simulink model "Filtro_teste_potencia_constante_burrice"  (R2014b)
settings: Solver=ode45  StartTime=0.0  StopTime=0.015  MaxStep=1e-6  RelTol=1e-5
libraries: powerlib x15, powerlib_meascontrol x2, powerlib_extras x1, dsparch4 x1
settings Model: Creator=JPSOLIV  LastModifiedBy=JPSOLIV

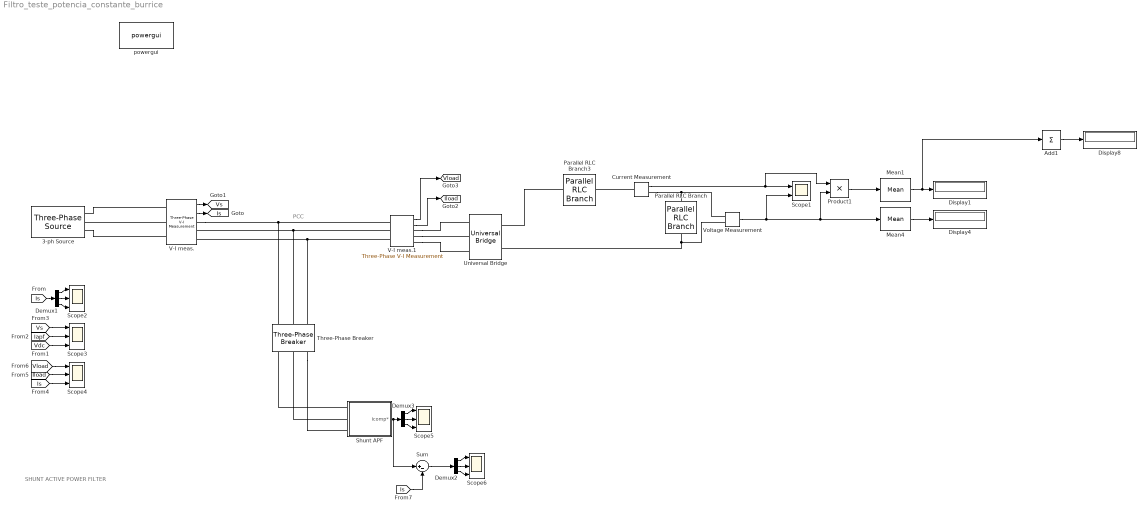
== system Filtro_teste_potencia_constante_burrice ==
  note: SHUNT ACTIVE POWER FILTER
  note: PCC
  3-ph Source : powerlib/Electrical Sources/Three-Phase Source  Voltage=115*sqrt(3)  PhaseAngle=0  Frequency=400  InternalConnection=Yg  SpecifyImpedance=off  Resistance=0.001  Inductance=1e-8  ShortCircuitLevel=100e6  BaseVoltage=25e3  XRratio=7  BusType=swing  Pref=0  Qref=0  Qmin=-inf  Qmax=inf
  Add1 : Sum  Inputs=+
  Current Measurement : powerlib/Measurements/Current Measurement  PhasorSimulation=off  OutputType=Complex  PSBequivalent=0
  Demux1 : Demux  Outputs=3
  Demux2 : Demux  Outputs=3
  Demux3 : Demux  Outputs=3
  Display1 : Display
  Display4 : Display
  Display8 : Display
  Mean1 : powerlib_meascontrol/Measurements/Mean  Freq=400  Vinit=0  Ts=0
  Mean4 : powerlib_meascontrol/Measurements/Mean  Freq=400  Vinit=0  Ts=0
  Parallel RLC Branch : powerlib/Elements/Parallel RLC Branch  LConnTagsString=a  RConnTagsString=__new0  BranchType=RC  Resistance=100  Inductance=1e-3  SetiL0=off  InitialCurrent=0  Capacitance=30e-6  Setx0=off  InitialVoltage=0  Measurements=None
  Parallel RLC Branch3 : powerlib/Elements/Parallel RLC Branch  LConnTagsString=a  RConnTagsString=__new0  BranchType=L  Resistance=1  Inductance=0.1e-3  SetiL0=off  InitialCurrent=0  Capacitance=30e-6  Setx0=off  InitialVoltage=0  Measurements=None
  Product1 : Product
  Scope1 : Scope  NumInputPorts=2
      settings: YMin=-20~0  YMax=160~600
  Scope{2..6} (5 alike) : Scope  NumInputPorts=3
      Scope2 settings: TimeRange=0.015  YMin=-2~-200~-50  YMax=12~50~200  SaveName=Isource  MaxDataPoints=500000
      Scope3 settings: TimeRange=0.015  YMin=-200~-10~-500  YMax=200~20~1500  SaveName=Vs_Iapf_Vdc  MaxDataPoints=500000
      Scope4 settings: TimeRange=0.015  YMin=-200~-200~-200  YMax=200~200~200  SaveName=Vs_Iapf_Vdc1  MaxDataPoints=500000
      Scope5 settings: TimeRange=0.015  YMin=-15~-50~-200  YMax=10~200~50  SaveName=Icomp  MaxDataPoints=500000
      Scope6 settings: TimeRange=0.015  YMin=-30~-30~-30  YMax=30~20~30  SaveName=Icomp1  MaxDataPoints=500000
  Shunt APF : Subsystem
  Sum : Sum  Inputs=|+-
  Three-Phase Breaker : powerlib/Elements/Three-Phase Breaker  InitialState=open  SwitchA=on  SwitchB=on  SwitchC=on  SwitchTimes=0.001  External=off  BreakerResistance=1e-6  SnubberResistance=1e6  SnubberCapacitance=inf  Measurements=None
  Universal Bridge : powerlib/Power Electronics/Universal Bridge  Arms=3  SnubberResistance=1e5  SnubberCapacitance=inf  Device=Diodes  Ron=1e-3  Lon=0  ForwardVoltages="[  0  0  ]"  ForwardVoltage=0  GTOparameters=[ 10e-6 , 20e-6 ]  IGBTparameters=[ 1e-6 , 2e-6 ]  Measurements=None  Measurements_2=None  converterType=Rectifier
  V-I meas. : powerlib/Measurements/Three-Phase V-I Measurement  VoltageMeasurement=phase-to-ground  SetLabelV=off  LabelV=Vabc  Vpu=off  VpuLL=off  CurrentMeasurement=yes  SetLabelI=off  LabelI=Iabc  Ipu=off  Pbase=100e6  Vbase=500e3  OutputType=Complex  PhasorSimulation=off  PSBequivalent=0
  V-I meas.1 : powerlib/Measurements/Three-Phase V-I Measurement  VoltageMeasurement=phase-to-ground  SetLabelV=off  LabelV=Vabc  Vpu=off  VpuLL=off  CurrentMeasurement=yes  SetLabelI=off  LabelI=Iabc  Ipu=off  Pbase=100e6  Vbase=500e3  OutputType=Complex  PhasorSimulation=off  PSBequivalent=0
  Voltage Measurement : powerlib/Measurements/Voltage Measurement  PhasorSimulation=off  OutputType=Complex  PSBequivalent=0
  powergui : powerlib/powergui  Priority=1  SimulationMode=Discrete  SolverType=Tustin/Backward Euler (TBE)  SampleTime=5e-6  frequency=60  SPID=off  DisableSnubberDevices=off  DisableRonSwitches=off  DisableVfSwitches=off  SwTol=0  DisplayEquations=off  Interpol=off  methode=off  Ts=100  frequencyindice=0  Pbase=100e6  ErrMax=1e-4  Iterations=50  UnitsV=kV  UnitsW=MW  FunctionMessages=off  echomessages=off  HookPort=off  EnableUseOfTLC=off  x0status=blocks  RestoreLinks=warning  ResistiveCurrentMeasurement=off  Frange=[0:2:500]  Ylog=off  Xlog=on  ShowGrid=off  save=off  variable=ZData  structure=psb3phPWM1_str8  ZoomFFT=off  StartTime=0.035  cycles=2  DisplayStyle=2  fundamental=50  FreqAxis=off  MaxFrequency=10000  frequencyindicesteady=1  RmsSteady=1  display=off
  tag scope: Iload=global, Is=global, Vload=global, Vs=global
  wires:
  Current Measurement/1 -> Product1/1, Scope1/1
  Voltage Measurement/1 -> Scope1/2, Product1/2, Mean4/1
  Product1/1 -> Mean1/1
  Mean1/1 -> Add1/1, Display1/1
  Mean4/1 -> Display4/1
  Add1/1 -> Display8/1
  V-I meas./1 -> [Vs]
  V-I meas./2 -> [Is]
  Demux3/1 -> Scope5/1
  Demux3/2 -> Scope5/2
  Demux3/3 -> Scope5/3
  Shunt APF/1(Icomp*) -> Sum/1, Demux3/1
  Demux1/1 -> Scope2/1
  Demux1/2 -> Scope2/2
  Demux1/3 -> Scope2/3
  [Is] -> Demux1/1
  [Vs] -> Scope3/1
  [Vdc] -> Scope3/3
  [Iapf] -> Scope3/2
  [Vload] -> Scope4/1
  [Is] -> Scope4/3
  [Iload] -> Scope4/2
  V-I meas.1/2 -> [Iload]
  V-I meas.1/1 -> [Vload]
  [Is] -> Sum/2
  Demux2/1 -> Scope6/1
  Demux2/2 -> Scope6/2
  Demux2/3 -> Scope6/3
  Sum/1 -> Demux2/1
  connections:
  Parallel RLC Branch/RConn1 -- Universal Bridge/RConn2 -- Voltage Measurement/LConn2
  Current Measurement/RConn1 -- Voltage Measurement/LConn1 -- Parallel RLC Branch/LConn1
  Parallel RLC Branch3/RConn1 -- Universal Bridge/RConn1
  Current Measurement/LConn1 -- Parallel RLC Branch3/LConn1
  V-I meas./RConn1 -- Three-Phase Breaker/LConn1 -- V-I meas.1/LConn1
  V-I meas.1/LConn3 -- Three-Phase Breaker/LConn3 -- V-I meas./RConn3
  3-ph Source/RConn3 -- V-I meas./LConn3
  V-I meas./LConn2 -- 3-ph Source/RConn2
  3-ph Source/RConn1 -- V-I meas./LConn1
  Shunt APF/LConn1 -- Three-Phase Breaker/RConn1
  Three-Phase Breaker/RConn3 -- Shunt APF/LConn3
  Shunt APF/LConn2 -- Three-Phase Breaker/RConn2
  V-I meas.1/LConn2 -- Three-Phase Breaker/LConn2 -- V-I meas./RConn2
  V-I meas.1/RConn1 -- Universal Bridge/LConn1
  V-I meas.1/RConn2 -- Universal Bridge/LConn2
  V-I meas.1/RConn3 -- Universal Bridge/LConn3

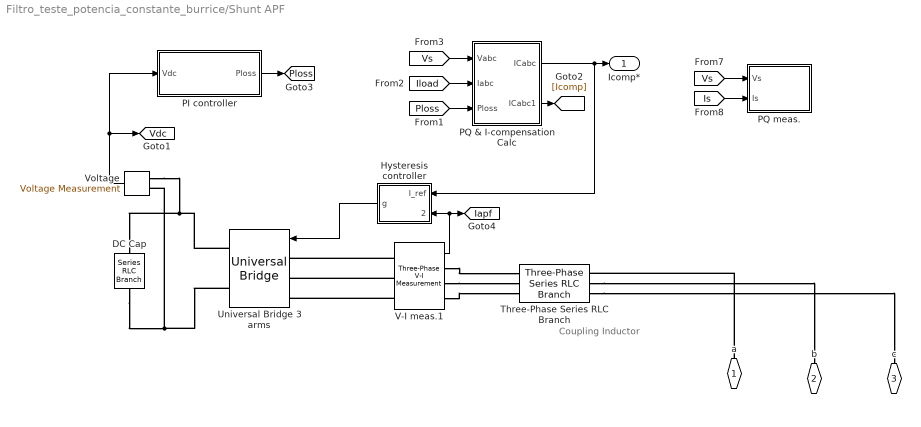
== system Filtro_teste_potencia_constante_burrice/Shunt APF ==
  note: Coupling Inductor
  DC Cap : powerlib/Elements/Series RLC Branch  LConnTagsString=__new0  RConnTagsString=__new0  BranchType=C  Resistance=1  Inductance=1e-3  SetiL0=off  InitialCurrent=0  Capacitance=3.5e-6  Setx0=off  InitialVoltage=400  Measurements=None
  Hysteresis controller : Subsystem
  PI controller : Subsystem
  PQ & I-compensation Calc : Subsystem
  PQ meas. : Subsystem
  Three-Phase Series RLC Branch : powerlib/Elements/Three-Phase Series RLC Branch  LConnTagsString=A|B|C  RConnTagsString=A|B|C  BranchType=L  Resistance=1e9  Inductance=10e-3  Capacitance=.2e-3  Measurements=None
  Universal Bridge 3 arms : powerlib/Power Electronics/Universal Bridge  Arms=3  SnubberResistance=10000  SnubberCapacitance=inf  Device=IGBT / Diodes  Ron=1e-4  Lon=0  ForwardVoltages="[  1  1  ]"  ForwardVoltage=.8  GTOparameters=[ 10e-6 , 20e-6 ]  IGBTparameters=[ 1e-6 , 2e-6 ]  Measurements=None  Measurements_2=None  converterType=Rectifier
  V-I meas.1 : powerlib/Measurements/Three-Phase V-I Measurement  VoltageMeasurement=phase-to-ground  SetLabelV=on  LabelV=Vnm  Vpu=off  VpuLL=off  CurrentMeasurement=yes  SetLabelI=off  LabelI=Iabc  Ipu=off  Pbase=100e6  Vbase=500e3  OutputType=Complex  PhasorSimulation=off  PSBequivalent=0
  Voltage : powerlib/Measurements/Voltage Measurement  PhasorSimulation=off  OutputType=Complex  PSBequivalent=0
  a : PMIOPort  Port=1  Side=Left
  b : PMIOPort  Port=2  Side=Left
  c : PMIOPort  Port=3  Side=Left
  Icomp* : Outport
  tag scope: Iapf=global, Ploss=global, Vdc=global
  wires:
  [Iload] -> PQ & I-compensation Calc/2(Iabc)
  V-I meas.1/1 -> Hysteresis controller/2(I_meas), [Iapf]
  Hysteresis controller/1(g) -> Universal Bridge 3 arms/1
  PQ & I-compensation Calc/1(ICabc) -> Hysteresis controller/1(I_ref), Icomp*/1
  Voltage/1 -> PI controller/1(Vdc), [Vdc]
  [Vs] -> PQ & I-compensation Calc/1(Vabc)
  PQ & I-compensation Calc/2(ICabc1) -> [Icomp]
  PI controller/1(Ploss) -> [Ploss]
  [Ploss] -> PQ & I-compensation Calc/3(Ploss)
  [Vs] -> PQ meas./1(Vs)
  [Is] -> PQ meas./2(Is)
  connections:
  Voltage/LConn1 -- DC Cap/LConn1 -- Universal Bridge 3 arms/RConn1
  V-I meas.1/LConn1 -- Universal Bridge 3 arms/LConn1
  V-I meas.1/LConn2 -- Universal Bridge 3 arms/LConn2
  V-I meas.1/RConn3 -- Three-Phase Series RLC Branch/LConn3
  V-I meas.1/RConn2 -- Three-Phase Series RLC Branch/LConn2
  V-I meas.1/LConn3 -- Universal Bridge 3 arms/LConn3
  V-I meas.1/RConn1 -- Three-Phase Series RLC Branch/LConn1
  a/RConn1 -- Three-Phase Series RLC Branch/RConn1
  Three-Phase Series RLC Branch/RConn2 -- b/RConn1
  Three-Phase Series RLC Branch/RConn3 -- c/RConn1
  DC Cap/RConn1 -- Universal Bridge 3 arms/RConn2 -- Voltage/LConn2

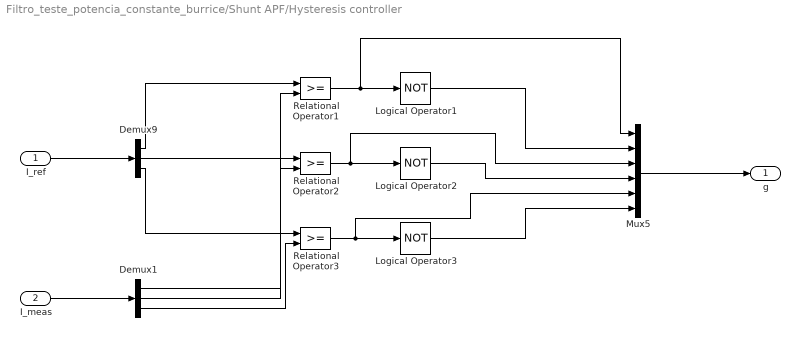
== system Filtro_teste_potencia_constante_burrice/Shunt APF/Hysteresis controller ==
  I_ref : Inport
  I_meas : Inport  Port=2
  Demux1 : Demux  Outputs=3
  Demux9 : Demux  Outputs=3
  Logical Operator1 : Logic  Operator=NOT  AllPortsSameDT=off  OutDataTypeStr=boolean
  Logical Operator2 : Logic  Operator=NOT  AllPortsSameDT=off  OutDataTypeStr=boolean
  Logical Operator3 : Logic  Operator=NOT  AllPortsSameDT=off  OutDataTypeStr=boolean
  Mux5 : Mux  Inputs=6
  Relational Operator1 : RelationalOperator  OutDataTypeStr=boolean
  Relational Operator2 : RelationalOperator  OutDataTypeStr=boolean
  Relational Operator3 : RelationalOperator  OutDataTypeStr=boolean
  g : Outport
  wires:
  Relational Operator1/1 -> Logical Operator1/1, Mux5/1
  Relational Operator2/1 -> Logical Operator2/1, Mux5/3
  Relational Operator3/1 -> Logical Operator3/1, Mux5/5
  Demux9/1 -> Relational Operator1/1
  Demux9/3 -> Relational Operator3/1
  Logical Operator1/1 -> Mux5/2
  Logical Operator2/1 -> Mux5/4
  Logical Operator3/1 -> Mux5/6
  Mux5/1 -> g/1
  Demux9/2 -> Relational Operator2/1
  Demux1/1 -> Relational Operator1/2
  Demux1/2 -> Relational Operator2/2
  Demux1/3 -> Relational Operator3/2
  I_ref/1 -> Demux9/1
  I_meas/1 -> Demux1/1

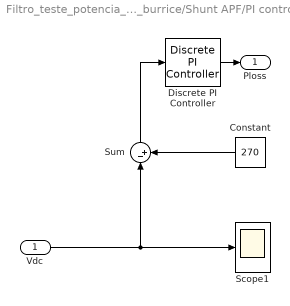
== system Filtro_teste_potencia_constante_burrice/Shunt APF/PI controller ==
  Vdc : Inport
  Constant : Constant  Value=270
  Discrete PI Controller : powerlib_extras/Discrete  Control Blocks/Discrete PI Controller  Kp=.1  Ki=1  Par_Limits=[1e6 -1e6]  Init=0  Ts=5e-6
  Scope1 : Scope
      settings: TimeRange=0.1  YMin=-20  YMax=140  SaveName=psb3phPWM1_str1  MaxDataPoints=500000
  Sum : Sum  Inputs=|-+
  Ploss : Outport
  wires:
  Constant/1 -> Sum/2
  Sum/1 -> Discrete PI Controller/1
  Discrete PI Controller/1 -> Ploss/1
  Vdc/1 -> Sum/1, Scope1/1

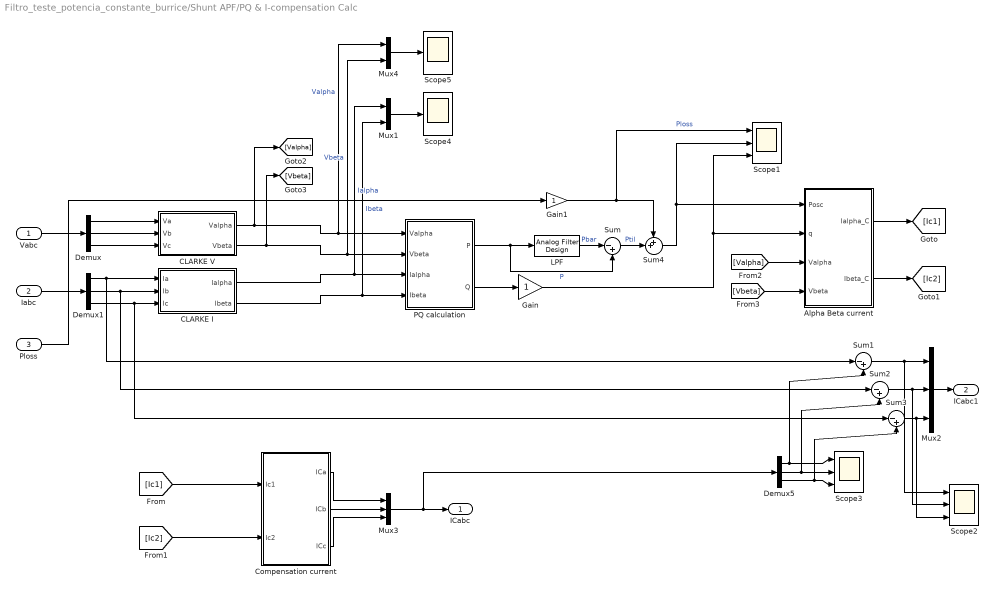
== system Filtro_teste_potencia_constante_burrice/Shunt APF/PQ & I-compensation Calc ==
  Vabc : Inport
  Iabc : Inport  Port=2
  Ploss : Inport  Port=3
  Alpha Beta current : MATLAB Function  TreatAsAtomicUnit=on
  CLARKE I : MATLAB Function  TreatAsAtomicUnit=on
  CLARKE V : MATLAB Function  TreatAsAtomicUnit=on
  Compensation current : MATLAB Function  TreatAsAtomicUnit=on
  Demux : Demux  Outputs=3
  Demux1 : Demux  Outputs=3
  Demux5 : Demux  Outputs=3
  Gain : Gain
  Gain1 : Gain
  LPF : dsparch4/Analog Filter Design  method=Butterworth  filttype=Lowpass  N=5  Wlo=2*pi*50  Whi=80  Rp=2  Rs=40
  Mux1 : Mux  Inputs=2
  Mux2 : Mux  Inputs=3
  Mux3 : Mux  Inputs=3
  Mux4 : Mux  Inputs=2
  PQ calculation : MATLAB Function  TreatAsAtomicUnit=on
  Scope1 : Scope  NumInputPorts=3
      settings: TimeRange=0.015  YMin=27~-50000~-12000  YMax=32~10000~2000  SaveName=psb3phPWM1_str9  MaxDataPoints=500000
  Scope2 : Scope  NumInputPorts=3
      settings: TimeRange=0.1  YMin=0.9825~-0.7725~-0.265  YMax=1.0025~-0.735~-0.21  SaveName=psb3phPWM1_str2  MaxDataPoints=500000
  Scope3 : Scope  NumInputPorts=3
      settings: TimeRange=0.1  YMin=-0.0625~-0.01~0.0325  YMax=-0.04~0.01~0.07  SaveName=psb3phPWM1_str7  MaxDataPoints=500000
  Scope4 : Scope
      settings: TimeRange=0.04  YMin=-200  YMax=200  SaveName=psb3phPWM1_str3  MaxDataPoints=500000
  Scope5 : Scope
      settings: TimeRange=0.015  YMin=-10  YMax=20  SaveName=psb3phPWM1_str4  MaxDataPoints=500000
  Sum{,1..3} (4 alike) : Sum  Inputs=|-+
  Sum4 : Sum  Inputs=++|
  ICabc : Outport
  ICabc1 : Outport  Port=2
  wires:
  Iabc/1 -> Demux1/1
  Vabc/1 -> Demux/1
  Compensation current/1(ICa) -> Mux3/1
  Compensation current/2(ICb) -> Mux3/2
  Compensation current/3(ICc) -> Mux3/3
  PQ calculation/2(Q) -> Gain/1
  PQ calculation/1(P) -> Sum/2, LPF/1  "P"
  Gain/1 -> Scope1/3, Alpha Beta current/2(q)
  Alpha Beta current/1(Ialpha_C) -> [Ic1]
  Alpha Beta current/2(Ibeta_C) -> [Ic2]
  Demux1/1 -> Sum1/1, CLARKE I/1(Ia)
  Gain1/1 -> Scope1/1, Sum4/1  "Ploss"
  Mux3/1 -> ICabc/1, Demux5/1
  Demux5/1 -> Scope3/1, Sum1/2
  Demux5/2 -> Scope3/2, Sum2/2
  Demux5/3 -> Scope3/3, Sum3/2
  Ploss/1 -> Gain1/1
  Sum1/1 -> Mux2/1, Scope2/1
  Sum2/1 -> Mux2/2, Scope2/2
  Sum3/1 -> Mux2/3, Scope2/3
  Mux2/1 -> ICabc1/1
  Demux/1 -> CLARKE V/1(Va)
  Demux1/2 -> CLARKE I/2(Ib), Sum2/1
  Demux1/3 -> CLARKE I/3(Ic), Sum3/1
  Demux/2 -> CLARKE V/2(Vb)
  Demux/3 -> CLARKE V/3(Vc)
  Mux1/1 -> Scope4/1
  Mux4/1 -> Scope5/1
  CLARKE V/1(Valpha) -> [Valpha], Mux4/1, PQ calculation/1(Valpha)  "Valpha"
  CLARKE V/2(Vbeta) -> [Vbeta], Mux4/2, PQ calculation/2(Vbeta)  "Vbeta"
  CLARKE I/1(Ialpha) -> Mux1/1, PQ calculation/3(Ialpha)  "Ialpha"
  CLARKE I/2(Ibeta) -> Mux1/2, PQ calculation/4(Ibeta)  "Ibeta"
  [Vbeta] -> Alpha Beta current/4(Vbeta)
  [Valpha] -> Alpha Beta current/3(Valpha)
  LPF/1 -> Sum/1  "Pbar"
  Sum/1 -> Sum4/2  "Ptil"
  Sum4/1 -> Alpha Beta current/1(Posc), Scope1/2
  [Ic1] -> Compensation current/1(Ic1)
  [Ic2] -> Compensation current/2(Ic2)

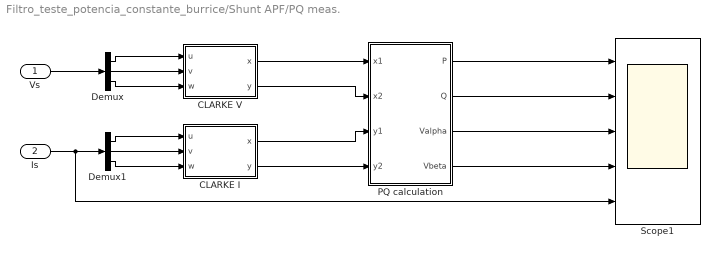
== system Filtro_teste_potencia_constante_burrice/Shunt APF/PQ meas. ==
  Vs : Inport
  Is : Inport  Port=2
  CLARKE I : MATLAB Function  TreatAsAtomicUnit=on
  CLARKE V : MATLAB Function  TreatAsAtomicUnit=on
  Demux : Demux  Outputs=3
  Demux1 : Demux  Outputs=3
  PQ calculation : MATLAB Function  TreatAsAtomicUnit=on
  Scope1 : Scope  NumInputPorts=5
      settings: TimeRange=0.1  YMin=49.75~-1~-39.955~-2.7~-1.25  YMax=51.5~1~-39.91~-1.8~0.75  SaveName=psb3phPWM1_str  MaxDataPoints=500000
  wires:
  CLARKE V/1(x) -> PQ calculation/1(x1)
  CLARKE V/2(y) -> PQ calculation/2(x2)
  CLARKE I/1(x) -> PQ calculation/3(y1)
  CLARKE I/2(y) -> PQ calculation/4(y2)
  Demux/1 -> CLARKE V/1(u)
  Demux/2 -> CLARKE V/2(v)
  Demux/3 -> CLARKE V/3(w)
  Demux1/1 -> CLARKE I/1(u)
  Demux1/2 -> CLARKE I/2(v)
  Demux1/3 -> CLARKE I/3(w)
  Vs/1 -> Demux/1
  Is/1 -> Demux1/1, Scope1/5
  PQ calculation/1(P) -> Scope1/1
  PQ calculation/2(Q) -> Scope1/2
  PQ calculation/3(Valpha) -> Scope1/3
  PQ calculation/4(Vbeta) -> Scope1/4

== matlab function Filtro_teste_potencia_constante_burrice/Shunt APF/PQ & I-compensation Calc/CLARKE I ==
  data: Ia input; Ialpha output; Ib input; Ic input; Ibeta output
function [Ialpha,Ibeta] = ICT(Ia,Ib,Ic)
%#em1

Ialpha = sqrt(2/3)*(Ia- 1/2*Ib - 1/2*Ic);
Ibeta = sqrt(2/3)*(0+ sqrt(3)/2*Ib - sqrt(3)/2*Ic);

== matlab function Filtro_teste_potencia_constante_burrice/Shunt APF/PQ & I-compensation Calc/CLARKE V ==
  data: Va input; Valpha output; Vb input; Vc input; Vbeta output
function [Valpha,Vbeta] = VCT(Va,Vb,Vc)
%#em1

Valpha = sqrt(2/3)*(Va - 1/2*Vb - 1/2*Vc);
Vbeta = sqrt(2/3)*(0 + sqrt(3)/2*Vb - sqrt(3)/2*Vc);

== matlab function Filtro_teste_potencia_constante_burrice/Shunt APF/PQ & I-compensation Calc/PQ calculation ==
  data: Valpha input; Vbeta input; Ialpha input; P output; Q output; Ibeta input
function [P,Q] = PQ(Valpha,Vbeta,Ialpha,Ibeta)
%#em1

P = (Valpha*Ialpha)+(Vbeta*Ibeta);
Q = (Vbeta*Ialpha)-(Valpha*Ibeta);

== matlab function Filtro_teste_potencia_constante_burrice/Shunt APF/PQ & I-compensation Calc/Compensation current ==
  data: Ic1 input; ICa output; Ic2 input; ICb output; ICc output
function [ICa,ICb,ICc] = Ical(Ic1,Ic2)
%#em1

ICa = sqrt(2/3)*(Ic1);
ICb = sqrt(2/3)*((-0.5*Ic1)+((sqrt(3)/2)*Ic2));
ICc = sqrt(2/3)*((-0.5*Ic1)-((sqrt(3)/2)*Ic2));

== matlab function Filtro_teste_potencia_constante_burrice/Shunt APF/PQ & I-compensation Calc/Alpha Beta current ==
  data: Posc input; Ialpha_C output; q input; Valpha input; Ibeta_C output; Vbeta input
function [Ialpha_C,Ibeta_C] = ICOM(Posc,q,Valpha,Vbeta)
%#em1

Ialpha_C = 1/(Valpha^2 + Vbeta^2)*(Posc*Valpha + q*Vbeta);
Ibeta_C = 1/(Valpha^2 + Vbeta^2)*(Posc*Vbeta - q*Valpha);

== matlab function Filtro_teste_potencia_constante_burrice/Shunt APF/PQ meas./CLARKE I ==
  data: u input; x output; v input; w input; y output
function [x,y] = ICT(u,v,w)
%#em1

x = sqrt(2/3)*(u-(0.5*v)-(0.5*w));
y = sqrt(2)*(0+(0.5*v)-(0.5*w));

== matlab function Filtro_teste_potencia_constante_burrice/Shunt APF/PQ meas./CLARKE V ==
  data: u input; x output; v input; w input; y output
function [x,y] = VCT(u,v,w)
%#em1

x = sqrt(2/3)*(u-(0.5*v)-(0.5*w));
y = sqrt(2)*(0+(0.5*v)-(0.5*w));

== matlab function Filtro_teste_potencia_constante_burrice/Shunt APF/PQ meas./PQ calculation ==
  data: x1 input; P output; Q output; x2 input; y1 input; y2 input; Valpha output; Vbeta output
function [P,Q,Valpha,Vbeta] = PQ(x1,x2,y1,y2)
%#em1

P = (x1*y1)+(x2*y2);
Q = (x2*y1)-(x1*y2);
Valpha = x1;
Vbeta = x2;
